simulink model "SecRwRtStLtwdRtwdTrgtPosSelc"  (R2018b)
settings: Solver=FixedStepDiscrete  StartTime=0.0  StopTime=10.0  FixedStep=0.01  RelTol=1e-3
undefined symbols (not defined in the file or in its folder): KeSMSw6sAcsEntrySecRwRtStLtwdRtwdPos_Val, KeSMSw6sAcsEntrySecRwRtStLtwdRtwdPosMax_Val, KeSMSw6sAcsEntrySecRwRtStLtwdRtwdPosMin_Val, KeSMSw6sAcsExtSecRwRtStLtwdRtwdPos_Val, KeSMSw6sAcsExtSecRwRtStLtwdRtwdPosMax_Val, KeSMSw6sAcsExtSecRwRtStLtwdRtwdPosMin_Val, KeSMSw6sFamilyMdSecRwRtStLtwdRtwdPos_Val, KeSMSw6sFamilyMdSecRwRtStLtwdRtwdPosMax_Val, KeSMSw6sFamilyMdSecRwRtStLtwdRtwdPosMin_Val, KeSMSw6sFamilyRMdSecRwRtStLtwdRtwdPos_Val, KeSMSw6sFamilyRMdSecRwRtStLtwdRtwdPosMax_Val, KeSMSw6sFamilyRMdSecRwRtStLtwdRtwdPosMin_Val, KeSMSw6sIntimacyMdSecRwRtStLtwdRtwdPos_Val, KeSMSw6sIntimacyMdSecRwRtStLtwdRtwdPosMax_Val, KeSMSw6sIntimacyMdSecRwRtStLtwdRtwdPosMin_Val, KeSMSw6sIntimacyRMdSecRwRtStLtwdRtwdPos_Val, KeSMSw6sIntimacyRMdSecRwRtStLtwdRtwdPosMax_Val, KeSMSw6sIntimacyRMdSecRwRtStLtwdRtwdPosMin_Val, KeSMSw6sVIPSecRwRtStLtwdRtwdPos_Val, KeSMSw6sVIPSecRwRtStLtwdRtwdPosMax_Val, KeSMSw6sVIPSecRwRtStLtwdRtwdPosMin_Val, KeSMSwAcsEntrySecRwRtStLtwdRtwdPos_Val, KeSMSwAcsEntrySecRwRtStLtwdRtwdPosMax_Val, KeSMSwAcsEntrySecRwRtStLtwdRtwdPosMin_Val, KeSMSwAcsExtSecRwRtStLtwdRtwdPos_Val, KeSMSwAcsExtSecRwRtStLtwdRtwdPosMax_Val, KeSMSwAcsExtSecRwRtStLtwdRtwdPosMin_Val, KeSMSwFamilyMdSecRwRtStLtwdRtwdPos_Val, KeSMSwFamilyMdSecRwRtStLtwdRtwdPosMax_Val, KeSMSwFamilyMdSecRwRtStLtwdRtwdPosMin_Val, KeSMSwFamilyRMdSecRwRtStLtwdRtwdPos_Val, KeSMSwFamilyRMdSecRwRtStLtwdRtwdPosMax_Val, KeSMSwFamilyRMdSecRwRtStLtwdRtwdPosMin_Val, KeSMSwIntimacyMdSecRwRtStLtwdRtwdPos_Val, KeSMSwIntimacyMdSecRwRtStLtwdRtwdPosMax_Val, KeSMSwIntimacyMdSecRwRtStLtwdRtwdPosMin_Val, KeSMSwIntimacyRMdSecRwRtStLtwdRtwdPos_Val, KeSMSwIntimacyRMdSecRwRtStLtwdRtwdPosMax_Val, KeSMSwIntimacyRMdSecRwRtStLtwdRtwdPosMin_Val, KeSMSwVIPSecRwRtStLtwdRtwdPos_Val, KeSMSwVIPSecRwRtStLtwdRtwdPosMax_Val, KeSMSwVIPSecRwRtStLtwdRtwdPosMin_Val
libraries: TrgtPosSelcLib x8
settings Model: Creator=sn2xws  LastModifiedBy=sn2xws
settings DataIOCC: SaveFormat=StructureWithTime
settings OptimizationCC: DefaultParameterBehavior=Inlined  EnhancedBackFolding=on  PassReuseOutputArgsAs=Individual arguments  ZeroExternalMemoryAtStartup=off  ZeroInternalMemoryAtStartup=off  OptimizeBlockOrder=speed  DifferentSizesBufferReuse=on  OptimizationCustomize=off
settings DebuggingCC: ParameterTunabilityLossMsg=error
settings ModelReferenceCC: ModelReferenceNumInstancesAllowed=Single
settings SFSimCC: MATLABDynamicMemAlloc=off
settings RTWCC: SystemTargetFile=autosar.tlc  GenCodeOnly=on  TemplateMakefile=ert_default_tmf  Description=AUTOSAR  GenerateReport=on  IncludeHyperlinkInReport=on  LaunchReport=on  GenerateTraceInfo=on  GenerateTraceReport=on  GenerateTraceReportSl=on  GenerateTraceReportSf=on  GenerateTraceReportEml=on
settings CodeAppCC: ForceParamTrailComments=on  IgnoreCustomStorageClasses=off  OperatorAnnotations=on  SimulinkDataObjDesc=on  SFDataObjDesc=on  InsertBlockDesc=on
settings STFCustomTargetCC: TargetLangStandard=C99 (ISO)  MultiwordLength=256  ParMdlRefBuildCompliant=on  CompOptLevelCompliant=on  IncludeMdlTerminateFcn=off  CombineOutputUpdateFcns=on  SuppressErrorStatus=on  ERTCustomFileBanners=on  SupportNonFinite=off  SupportComplex=off  SupportContinuousTime=off  SupportNonInlinedSFcns=off  RemoveResetFunc=on  MATLABClassNameForMDSCustomization=Simulink.SoftwareTarget.ERTCustomization  AutosarCompliant=on  UseToolchainInfoCompliant=on  LookupTableObjectStructAxisOrder=2,1,3,4,...  LUTObjectStructOrderEvenSpacing=Size,Table,Breakpoints  SystemTargetFile=autosar.tlc
settings ERTTargetCC: TargetLangStandard=C99 (ISO)  ConcurrentExecutionCompliant=off  IncludeMdlTerminateFcn=off  SuppressErrorStatus=on  SupportNonFinite=off  SupportComplex=off  ModelStepFunctionPrototypeControlCompliant=off  CPPClassGenCompliant=off  AutosarCompliant=on  LookupTableObjectStructAxisOrder=2,1,3,4,...  LUTObjectStructOrderEvenSpacing=Size,Table,Breakpoints  InlinedParameterPlacement=NonHierarchical  ERTCustomFileTemplate=example_file_process.tlc  ERTFilePackagingFormat=Compact

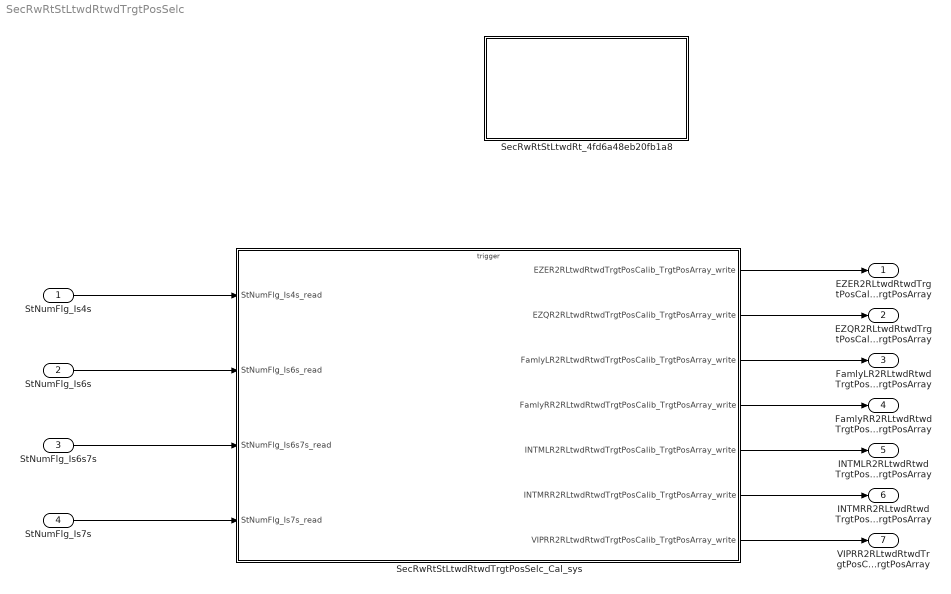
== system SecRwRtStLtwdRtwdTrgtPosSelc ==
  StNumFlg_Is4s : Inport  OutDataTypeStr=boolean  PortDimensions=1
  StNumFlg_Is6s : Inport  Port=2  OutDataTypeStr=boolean  PortDimensions=1
  StNumFlg_Is6s7s : Inport  Port=3  OutDataTypeStr=boolean  PortDimensions=1
  StNumFlg_Is7s : Inport  Port=4  OutDataTypeStr=boolean  PortDimensions=1
  SecRwRtStLtwdRt_4fd6a48eb20fb1a8 : Subsystem
  SecRwRtStLtwdRtwdTrgtPosSelc_Cal_sys : Subsystem
  EZER2RLtwdRtwdTrgtPosCalib_TrgtPosArray : Outport  Description=|  OutDataTypeStr=uint16  PortDimensions=3
      | 0:Pos
      | 1:Max
      | 2:Min
  EZQR2RLtwdRtwdTrgtPosCalib_TrgtPosArray : Outport  Description=|  Port=2  OutDataTypeStr=uint16  PortDimensions=3
      | 0:Pos
      | 1:Max
      | 2:Min
  FamlyLR2RLtwdRtwdTrgtPosCalib_TrgtPosArray : Outport  Description=|  Port=3  OutDataTypeStr=uint16  PortDimensions=3
      | 0:Pos
      | 1:Max
      | 2:Min
  FamlyRR2RLtwdRtwdTrgtPosCalib_TrgtPosArray : Outport  Description=|  Port=4  OutDataTypeStr=uint16  PortDimensions=3
      | 0:Pos
      | 1:Max
      | 2:Min
  INTMLR2RLtwdRtwdTrgtPosCalib_TrgtPosArray : Outport  Description=|  Port=5  OutDataTypeStr=uint16  PortDimensions=3
      | 0:Pos
      | 1:Max
      | 2:Min
  INTMRR2RLtwdRtwdTrgtPosCalib_TrgtPosArray : Outport  Description=|  Port=6  OutDataTypeStr=uint16  PortDimensions=3
      | 0:Pos
      | 1:Max
      | 2:Min
  VIPRR2RLtwdRtwdTrgtPosCalib_TrgtPosArray : Outport  Description=|  Port=7  OutDataTypeStr=uint16  PortDimensions=3
      | 0:Pos
      | 1:Max
      | 2:Min
  wires:
  StNumFlg_Is4s/1 -> SecRwRtStLtwdRtwdTrgtPosSelc_Cal_sys/1(StNumFlg_Is4s_read)
  StNumFlg_Is6s/1 -> SecRwRtStLtwdRtwdTrgtPosSelc_Cal_sys/2(StNumFlg_Is6s_read)
  StNumFlg_Is6s7s/1 -> SecRwRtStLtwdRtwdTrgtPosSelc_Cal_sys/3(StNumFlg_Is6s7s_read)
  StNumFlg_Is7s/1 -> SecRwRtStLtwdRtwdTrgtPosSelc_Cal_sys/4(StNumFlg_Is7s_read)
  SecRwRtStLtwdRtwdTrgtPosSelc_Cal_sys/1(EZER2RLtwdRtwdTrgtPosCalib_TrgtPosArray_write) -> EZER2RLtwdRtwdTrgtPosCalib_TrgtPosArray/1
  SecRwRtStLtwdRtwdTrgtPosSelc_Cal_sys/2(EZQR2RLtwdRtwdTrgtPosCalib_TrgtPosArray_write) -> EZQR2RLtwdRtwdTrgtPosCalib_TrgtPosArray/1
  SecRwRtStLtwdRtwdTrgtPosSelc_Cal_sys/3(FamlyLR2RLtwdRtwdTrgtPosCalib_TrgtPosArray_write) -> FamlyLR2RLtwdRtwdTrgtPosCalib_TrgtPosArray/1
  SecRwRtStLtwdRtwdTrgtPosSelc_Cal_sys/4(FamlyRR2RLtwdRtwdTrgtPosCalib_TrgtPosArray_write) -> FamlyRR2RLtwdRtwdTrgtPosCalib_TrgtPosArray/1
  SecRwRtStLtwdRtwdTrgtPosSelc_Cal_sys/5(INTMLR2RLtwdRtwdTrgtPosCalib_TrgtPosArray_write) -> INTMLR2RLtwdRtwdTrgtPosCalib_TrgtPosArray/1
  SecRwRtStLtwdRtwdTrgtPosSelc_Cal_sys/6(INTMRR2RLtwdRtwdTrgtPosCalib_TrgtPosArray_write) -> INTMRR2RLtwdRtwdTrgtPosCalib_TrgtPosArray/1
  SecRwRtStLtwdRtwdTrgtPosSelc_Cal_sys/7(VIPRR2RLtwdRtwdTrgtPosCalib_TrgtPosArray_write) -> VIPRR2RLtwdRtwdTrgtPosCalib_TrgtPosArray/1

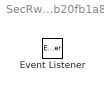
== system SecRwRtStLtwdRtwdTrgtPosSelc/SecRwRtStLtwdRt_4fd6a48eb20fb1a8 ==
  Event Listener : EventListener  EventName=reset

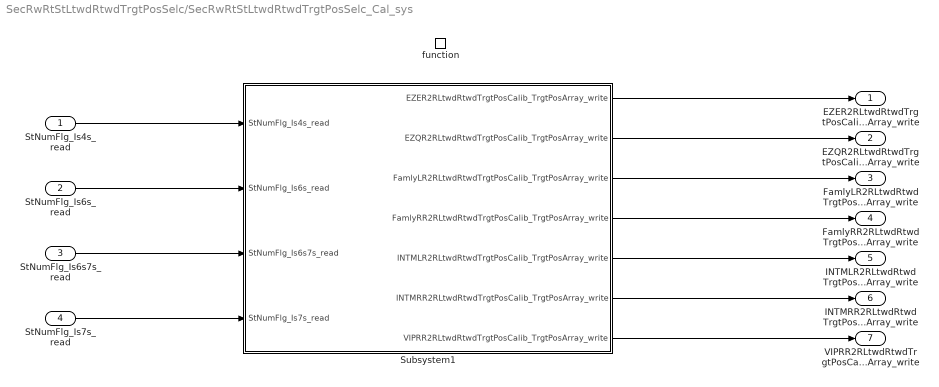
== system SecRwRtStLtwdRtwdTrgtPosSelc/SecRwRtStLtwdRtwdTrgtPosSelc_Cal_sys ==
  StNumFlg_Is4s_read : Inport
  StNumFlg_Is6s_read : Inport  Port=2
  StNumFlg_Is6s7s_read : Inport  Port=3
  StNumFlg_Is7s_read : Inport  Port=4
  function : TriggerPort  TriggerType=function-call  IsSimulinkFunction=on  FunctionName=SecRwRtStLtwdRtwdTrgtPosSelc_Cal  VariantControl=(inherit)
  Subsystem1 : Subsystem
  EZER2RLtwdRtwdTrgtPosCalib_TrgtPosArray_write : Outport
      settings: EnsureOutportIsVirtual=on
  EZQR2RLtwdRtwdTrgtPosCalib_TrgtPosArray_write : Outport  Port=2
      settings: EnsureOutportIsVirtual=on
  FamlyLR2RLtwdRtwdTrgtPosCalib_TrgtPosArray_write : Outport  Port=3
      settings: EnsureOutportIsVirtual=on
  FamlyRR2RLtwdRtwdTrgtPosCalib_TrgtPosArray_write : Outport  Port=4
      settings: EnsureOutportIsVirtual=on
  INTMLR2RLtwdRtwdTrgtPosCalib_TrgtPosArray_write : Outport  Port=5
      settings: EnsureOutportIsVirtual=on
  INTMRR2RLtwdRtwdTrgtPosCalib_TrgtPosArray_write : Outport  Port=6
      settings: EnsureOutportIsVirtual=on
  VIPRR2RLtwdRtwdTrgtPosCalib_TrgtPosArray_write : Outport  Port=7
      settings: EnsureOutportIsVirtual=on
  wires:
  Subsystem1/1(EZER2RLtwdRtwdTrgtPosCalib_TrgtPosArray_write) -> EZER2RLtwdRtwdTrgtPosCalib_TrgtPosArray_write/1
  Subsystem1/2(EZQR2RLtwdRtwdTrgtPosCalib_TrgtPosArray_write) -> EZQR2RLtwdRtwdTrgtPosCalib_TrgtPosArray_write/1
  Subsystem1/3(FamlyLR2RLtwdRtwdTrgtPosCalib_TrgtPosArray_write) -> FamlyLR2RLtwdRtwdTrgtPosCalib_TrgtPosArray_write/1
  Subsystem1/4(FamlyRR2RLtwdRtwdTrgtPosCalib_TrgtPosArray_write) -> FamlyRR2RLtwdRtwdTrgtPosCalib_TrgtPosArray_write/1
  Subsystem1/5(INTMLR2RLtwdRtwdTrgtPosCalib_TrgtPosArray_write) -> INTMLR2RLtwdRtwdTrgtPosCalib_TrgtPosArray_write/1
  Subsystem1/6(INTMRR2RLtwdRtwdTrgtPosCalib_TrgtPosArray_write) -> INTMRR2RLtwdRtwdTrgtPosCalib_TrgtPosArray_write/1
  Subsystem1/7(VIPRR2RLtwdRtwdTrgtPosCalib_TrgtPosArray_write) -> VIPRR2RLtwdRtwdTrgtPosCalib_TrgtPosArray_write/1
  StNumFlg_Is4s_read/1 -> Subsystem1/1(StNumFlg_Is4s_read)
  StNumFlg_Is6s_read/1 -> Subsystem1/2(StNumFlg_Is6s_read)
  StNumFlg_Is6s7s_read/1 -> Subsystem1/3(StNumFlg_Is6s7s_read)
  StNumFlg_Is7s_read/1 -> Subsystem1/4(StNumFlg_Is7s_read)

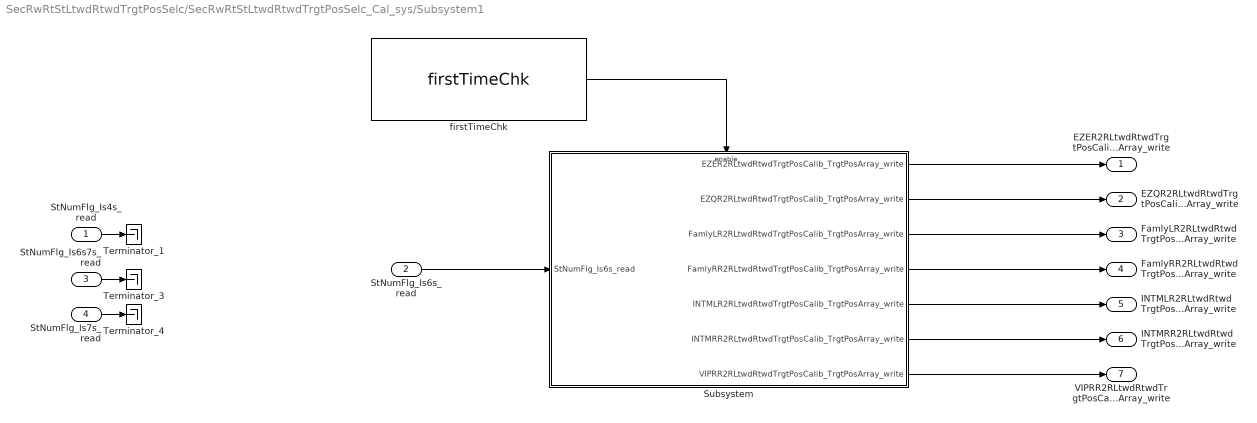
== system SecRwRtStLtwdRtwdTrgtPosSelc/SecRwRtStLtwdRtwdTrgtPosSelc_Cal_sys/Subsystem1 ==
  StNumFlg_Is4s_read : Inport
  StNumFlg_Is6s_read : Inport  Port=2
  StNumFlg_Is6s7s_read : Inport  Port=3
  StNumFlg_Is7s_read : Inport  Port=4
  Subsystem : Subsystem
  Terminator_1 : Terminator
  Terminator_3 : Terminator
  Terminator_4 : Terminator
  firstTimeChk : TrgtPosSelcLib/firstTimeChk  SystemSampleTime=-1
  EZER2RLtwdRtwdTrgtPosCalib_TrgtPosArray_write : Outport
      settings: EnsureOutportIsVirtual=on
  EZQR2RLtwdRtwdTrgtPosCalib_TrgtPosArray_write : Outport  Port=2
      settings: EnsureOutportIsVirtual=on
  FamlyLR2RLtwdRtwdTrgtPosCalib_TrgtPosArray_write : Outport  Port=3
      settings: EnsureOutportIsVirtual=on
  FamlyRR2RLtwdRtwdTrgtPosCalib_TrgtPosArray_write : Outport  Port=4
      settings: EnsureOutportIsVirtual=on
  INTMLR2RLtwdRtwdTrgtPosCalib_TrgtPosArray_write : Outport  Port=5
      settings: EnsureOutportIsVirtual=on
  INTMRR2RLtwdRtwdTrgtPosCalib_TrgtPosArray_write : Outport  Port=6
      settings: EnsureOutportIsVirtual=on
  VIPRR2RLtwdRtwdTrgtPosCalib_TrgtPosArray_write : Outport  Port=7
      settings: EnsureOutportIsVirtual=on
  wires:
  Subsystem/2(EZQR2RLtwdRtwdTrgtPosCalib_TrgtPosArray_write) -> EZQR2RLtwdRtwdTrgtPosCalib_TrgtPosArray_write/1
  StNumFlg_Is6s_read/1 -> Subsystem/1(StNumFlg_Is6s_read)
  StNumFlg_Is6s7s_read/1 -> Terminator_3/1
  firstTimeChk/1 -> Subsystem/Enable
  Subsystem/1(EZER2RLtwdRtwdTrgtPosCalib_TrgtPosArray_write) -> EZER2RLtwdRtwdTrgtPosCalib_TrgtPosArray_write/1
  StNumFlg_Is7s_read/1 -> Terminator_4/1
  Subsystem/3(FamlyLR2RLtwdRtwdTrgtPosCalib_TrgtPosArray_write) -> FamlyLR2RLtwdRtwdTrgtPosCalib_TrgtPosArray_write/1
  Subsystem/4(FamlyRR2RLtwdRtwdTrgtPosCalib_TrgtPosArray_write) -> FamlyRR2RLtwdRtwdTrgtPosCalib_TrgtPosArray_write/1
  Subsystem/5(INTMLR2RLtwdRtwdTrgtPosCalib_TrgtPosArray_write) -> INTMLR2RLtwdRtwdTrgtPosCalib_TrgtPosArray_write/1
  Subsystem/7(VIPRR2RLtwdRtwdTrgtPosCalib_TrgtPosArray_write) -> VIPRR2RLtwdRtwdTrgtPosCalib_TrgtPosArray_write/1
  StNumFlg_Is4s_read/1 -> Terminator_1/1
  Subsystem/6(INTMRR2RLtwdRtwdTrgtPosCalib_TrgtPosArray_write) -> INTMRR2RLtwdRtwdTrgtPosCalib_TrgtPosArray_write/1

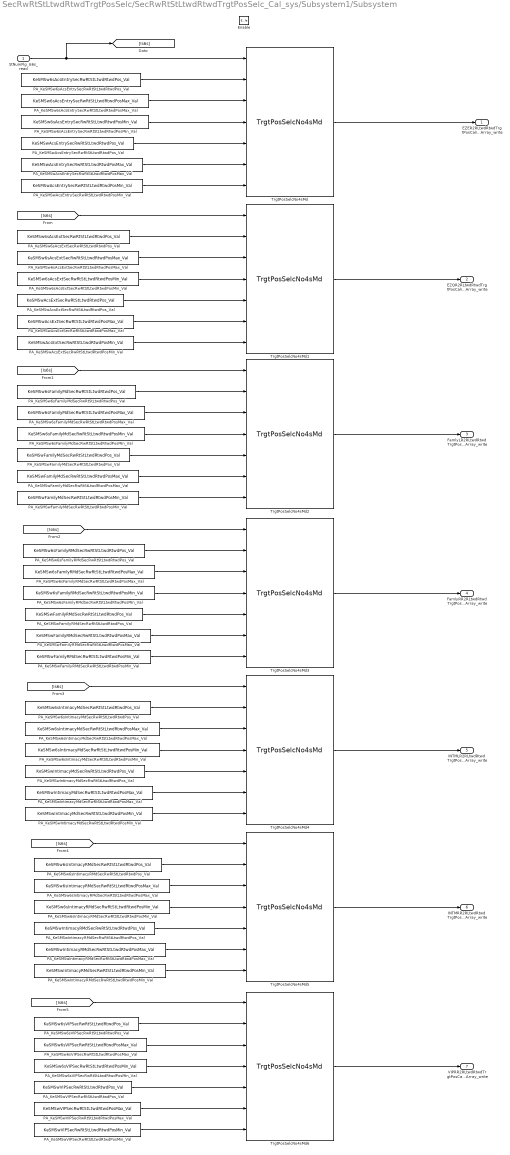
== system SecRwRtStLtwdRtwdTrgtPosSelc/SecRwRtStLtwdRtwdTrgtPosSelc_Cal_sys/Subsystem1/Subsystem ==
  StNumFlg_Is6s_read : Inport
  Enable : EnablePort
  PA_KeSMSw6sAcsEntrySecRwRtStLtwdRtwdPosMax_Val : Constant  Value=KeSMSw6sAcsEntrySecRwRtStLtwdRtwdPosMax_Val
  PA_KeSMSw6sAcsEntrySecRwRtStLtwdRtwdPosMin_Val : Constant  Value=KeSMSw6sAcsEntrySecRwRtStLtwdRtwdPosMin_Val
  PA_KeSMSw6sAcsEntrySecRwRtStLtwdRtwdPos_Val : Constant  Value=KeSMSw6sAcsEntrySecRwRtStLtwdRtwdPos_Val
  PA_KeSMSw6sAcsExtSecRwRtStLtwdRtwdPosMax_Val : Constant  Value=KeSMSw6sAcsExtSecRwRtStLtwdRtwdPosMax_Val
  PA_KeSMSw6sAcsExtSecRwRtStLtwdRtwdPosMin_Val : Constant  Value=KeSMSw6sAcsExtSecRwRtStLtwdRtwdPosMin_Val
  PA_KeSMSw6sAcsExtSecRwRtStLtwdRtwdPos_Val : Constant  Value=KeSMSw6sAcsExtSecRwRtStLtwdRtwdPos_Val
  PA_KeSMSw6sFamilyMdSecRwRtStLtwdRtwdPosMax_Val : Constant  Value=KeSMSw6sFamilyMdSecRwRtStLtwdRtwdPosMax_Val
  PA_KeSMSw6sFamilyMdSecRwRtStLtwdRtwdPosMin_Val : Constant  Value=KeSMSw6sFamilyMdSecRwRtStLtwdRtwdPosMin_Val
  PA_KeSMSw6sFamilyMdSecRwRtStLtwdRtwdPos_Val : Constant  Value=KeSMSw6sFamilyMdSecRwRtStLtwdRtwdPos_Val
  PA_KeSMSw6sFamilyRMdSecRwRtStLtwdRtwdPosMax_Val : Constant  Value=KeSMSw6sFamilyRMdSecRwRtStLtwdRtwdPosMax_Val
  PA_KeSMSw6sFamilyRMdSecRwRtStLtwdRtwdPosMin_Val : Constant  Value=KeSMSw6sFamilyRMdSecRwRtStLtwdRtwdPosMin_Val
  PA_KeSMSw6sFamilyRMdSecRwRtStLtwdRtwdPos_Val : Constant  Value=KeSMSw6sFamilyRMdSecRwRtStLtwdRtwdPos_Val
  PA_KeSMSw6sIntimacyMdSecRwRtStLtwdRtwdPosMax_Val : Constant  Value=KeSMSw6sIntimacyMdSecRwRtStLtwdRtwdPosMax_Val
  PA_KeSMSw6sIntimacyMdSecRwRtStLtwdRtwdPosMin_Val : Constant  Value=KeSMSw6sIntimacyMdSecRwRtStLtwdRtwdPosMin_Val
  PA_KeSMSw6sIntimacyMdSecRwRtStLtwdRtwdPos_Val : Constant  Value=KeSMSw6sIntimacyMdSecRwRtStLtwdRtwdPos_Val
  PA_KeSMSw6sIntimacyRMdSecRwRtStLtwdRtwdPosMax_Val : Constant  Value=KeSMSw6sIntimacyRMdSecRwRtStLtwdRtwdPosMax_Val
  PA_KeSMSw6sIntimacyRMdSecRwRtStLtwdRtwdPosMin_Val : Constant  Value=KeSMSw6sIntimacyRMdSecRwRtStLtwdRtwdPosMin_Val
  PA_KeSMSw6sIntimacyRMdSecRwRtStLtwdRtwdPos_Val : Constant  Value=KeSMSw6sIntimacyRMdSecRwRtStLtwdRtwdPos_Val
  PA_KeSMSw6sVIPSecRwRtStLtwdRtwdPosMax_Val : Constant  Value=KeSMSw6sVIPSecRwRtStLtwdRtwdPosMax_Val
  PA_KeSMSw6sVIPSecRwRtStLtwdRtwdPosMin_Val : Constant  Value=KeSMSw6sVIPSecRwRtStLtwdRtwdPosMin_Val
  PA_KeSMSw6sVIPSecRwRtStLtwdRtwdPos_Val : Constant  Value=KeSMSw6sVIPSecRwRtStLtwdRtwdPos_Val
  PA_KeSMSwAcsEntrySecRwRtStLtwdRtwdPosMax_Val : Constant  Value=KeSMSwAcsEntrySecRwRtStLtwdRtwdPosMax_Val
  PA_KeSMSwAcsEntrySecRwRtStLtwdRtwdPosMin_Val : Constant  Value=KeSMSwAcsEntrySecRwRtStLtwdRtwdPosMin_Val
  PA_KeSMSwAcsEntrySecRwRtStLtwdRtwdPos_Val : Constant  Value=KeSMSwAcsEntrySecRwRtStLtwdRtwdPos_Val
  PA_KeSMSwAcsExtSecRwRtStLtwdRtwdPosMax_Val : Constant  Value=KeSMSwAcsExtSecRwRtStLtwdRtwdPosMax_Val
  PA_KeSMSwAcsExtSecRwRtStLtwdRtwdPosMin_Val : Constant  Value=KeSMSwAcsExtSecRwRtStLtwdRtwdPosMin_Val
  PA_KeSMSwAcsExtSecRwRtStLtwdRtwdPos_Val : Constant  Value=KeSMSwAcsExtSecRwRtStLtwdRtwdPos_Val
  PA_KeSMSwFamilyMdSecRwRtStLtwdRtwdPosMax_Val : Constant  Value=KeSMSwFamilyMdSecRwRtStLtwdRtwdPosMax_Val
  PA_KeSMSwFamilyMdSecRwRtStLtwdRtwdPosMin_Val : Constant  Value=KeSMSwFamilyMdSecRwRtStLtwdRtwdPosMin_Val
  PA_KeSMSwFamilyMdSecRwRtStLtwdRtwdPos_Val : Constant  Value=KeSMSwFamilyMdSecRwRtStLtwdRtwdPos_Val
  PA_KeSMSwFamilyRMdSecRwRtStLtwdRtwdPosMax_Val : Constant  Value=KeSMSwFamilyRMdSecRwRtStLtwdRtwdPosMax_Val
  PA_KeSMSwFamilyRMdSecRwRtStLtwdRtwdPosMin_Val : Constant  Value=KeSMSwFamilyRMdSecRwRtStLtwdRtwdPosMin_Val
  PA_KeSMSwFamilyRMdSecRwRtStLtwdRtwdPos_Val : Constant  Value=KeSMSwFamilyRMdSecRwRtStLtwdRtwdPos_Val
  PA_KeSMSwIntimacyMdSecRwRtStLtwdRtwdPosMax_Val : Constant  Value=KeSMSwIntimacyMdSecRwRtStLtwdRtwdPosMax_Val
  PA_KeSMSwIntimacyMdSecRwRtStLtwdRtwdPosMin_Val : Constant  Value=KeSMSwIntimacyMdSecRwRtStLtwdRtwdPosMin_Val
  PA_KeSMSwIntimacyMdSecRwRtStLtwdRtwdPos_Val : Constant  Value=KeSMSwIntimacyMdSecRwRtStLtwdRtwdPos_Val
  PA_KeSMSwIntimacyRMdSecRwRtStLtwdRtwdPosMax_Val : Constant  Value=KeSMSwIntimacyRMdSecRwRtStLtwdRtwdPosMax_Val
  PA_KeSMSwIntimacyRMdSecRwRtStLtwdRtwdPosMin_Val : Constant  Value=KeSMSwIntimacyRMdSecRwRtStLtwdRtwdPosMin_Val
  PA_KeSMSwIntimacyRMdSecRwRtStLtwdRtwdPos_Val : Constant  Value=KeSMSwIntimacyRMdSecRwRtStLtwdRtwdPos_Val
  PA_KeSMSwVIPSecRwRtStLtwdRtwdPosMax_Val : Constant  Value=KeSMSwVIPSecRwRtStLtwdRtwdPosMax_Val
  PA_KeSMSwVIPSecRwRtStLtwdRtwdPosMin_Val : Constant  Value=KeSMSwVIPSecRwRtStLtwdRtwdPosMin_Val
  PA_KeSMSwVIPSecRwRtStLtwdRtwdPos_Val : Constant  Value=KeSMSwVIPSecRwRtStLtwdRtwdPos_Val
  TrgtPosSelcNo4sMd{,1..6} (7 alike) : TrgtPosSelcLib/TrgtPosSelcNo4sMd  SystemSampleTime=-1
  EZER2RLtwdRtwdTrgtPosCalib_TrgtPosArray_write : Outport
      settings: EnsureOutportIsVirtual=on
  EZQR2RLtwdRtwdTrgtPosCalib_TrgtPosArray_write : Outport  Port=2
      settings: EnsureOutportIsVirtual=on
  FamlyLR2RLtwdRtwdTrgtPosCalib_TrgtPosArray_write : Outport  Port=3
      settings: EnsureOutportIsVirtual=on
  FamlyRR2RLtwdRtwdTrgtPosCalib_TrgtPosArray_write : Outport  Port=4
      settings: EnsureOutportIsVirtual=on
  INTMLR2RLtwdRtwdTrgtPosCalib_TrgtPosArray_write : Outport  Port=5
      settings: EnsureOutportIsVirtual=on
  INTMRR2RLtwdRtwdTrgtPosCalib_TrgtPosArray_write : Outport  Port=6
      settings: EnsureOutportIsVirtual=on
  VIPRR2RLtwdRtwdTrgtPosCalib_TrgtPosArray_write : Outport  Port=7
      settings: EnsureOutportIsVirtual=on
  wires:
  TrgtPosSelcNo4sMd/1 -> EZER2RLtwdRtwdTrgtPosCalib_TrgtPosArray_write/1
  TrgtPosSelcNo4sMd1/1 -> EZQR2RLtwdRtwdTrgtPosCalib_TrgtPosArray_write/1
  StNumFlg_Is6s_read/1 -> [Is6s], TrgtPosSelcNo4sMd/1
  [Is6s] -> TrgtPosSelcNo4sMd1/1
  [Is6s] -> TrgtPosSelcNo4sMd2/1
  [Is6s] -> TrgtPosSelcNo4sMd3/1
  [Is6s] -> TrgtPosSelcNo4sMd4/1
  [Is6s] -> TrgtPosSelcNo4sMd5/1
  [Is6s] -> TrgtPosSelcNo4sMd6/1
  TrgtPosSelcNo4sMd2/1 -> FamlyLR2RLtwdRtwdTrgtPosCalib_TrgtPosArray_write/1
  TrgtPosSelcNo4sMd3/1 -> FamlyRR2RLtwdRtwdTrgtPosCalib_TrgtPosArray_write/1
  TrgtPosSelcNo4sMd4/1 -> INTMLR2RLtwdRtwdTrgtPosCalib_TrgtPosArray_write/1
  TrgtPosSelcNo4sMd5/1 -> INTMRR2RLtwdRtwdTrgtPosCalib_TrgtPosArray_write/1
  TrgtPosSelcNo4sMd6/1 -> VIPRR2RLtwdRtwdTrgtPosCalib_TrgtPosArray_write/1
  PA_KeSMSw6sAcsEntrySecRwRtStLtwdRtwdPosMax_Val/1 -> TrgtPosSelcNo4sMd/3
  PA_KeSMSw6sAcsEntrySecRwRtStLtwdRtwdPos_Val/1 -> TrgtPosSelcNo4sMd/2
  PA_KeSMSw6sAcsEntrySecRwRtStLtwdRtwdPosMin_Val/1 -> TrgtPosSelcNo4sMd/4
  PA_KeSMSw6sAcsExtSecRwRtStLtwdRtwdPosMax_Val/1 -> TrgtPosSelcNo4sMd1/3
  PA_KeSMSw6sAcsExtSecRwRtStLtwdRtwdPos_Val/1 -> TrgtPosSelcNo4sMd1/2
  PA_KeSMSw6sAcsExtSecRwRtStLtwdRtwdPosMin_Val/1 -> TrgtPosSelcNo4sMd1/4
  PA_KeSMSw6sFamilyMdSecRwRtStLtwdRtwdPosMax_Val/1 -> TrgtPosSelcNo4sMd2/3
  PA_KeSMSw6sFamilyMdSecRwRtStLtwdRtwdPos_Val/1 -> TrgtPosSelcNo4sMd2/2
  PA_KeSMSw6sFamilyMdSecRwRtStLtwdRtwdPosMin_Val/1 -> TrgtPosSelcNo4sMd2/4
  PA_KeSMSw6sFamilyRMdSecRwRtStLtwdRtwdPosMax_Val/1 -> TrgtPosSelcNo4sMd3/3
  PA_KeSMSw6sFamilyRMdSecRwRtStLtwdRtwdPos_Val/1 -> TrgtPosSelcNo4sMd3/2
  PA_KeSMSw6sFamilyRMdSecRwRtStLtwdRtwdPosMin_Val/1 -> TrgtPosSelcNo4sMd3/4
  PA_KeSMSw6sIntimacyMdSecRwRtStLtwdRtwdPosMax_Val/1 -> TrgtPosSelcNo4sMd4/3
  PA_KeSMSw6sIntimacyMdSecRwRtStLtwdRtwdPosMin_Val/1 -> TrgtPosSelcNo4sMd4/4
  PA_KeSMSw6sIntimacyMdSecRwRtStLtwdRtwdPos_Val/1 -> TrgtPosSelcNo4sMd4/2
  PA_KeSMSw6sIntimacyRMdSecRwRtStLtwdRtwdPosMin_Val/1 -> TrgtPosSelcNo4sMd5/4
  PA_KeSMSw6sIntimacyRMdSecRwRtStLtwdRtwdPosMax_Val/1 -> TrgtPosSelcNo4sMd5/3
  PA_KeSMSw6sIntimacyRMdSecRwRtStLtwdRtwdPos_Val/1 -> TrgtPosSelcNo4sMd5/2
  PA_KeSMSw6sVIPSecRwRtStLtwdRtwdPosMax_Val/1 -> TrgtPosSelcNo4sMd6/3
  PA_KeSMSw6sVIPSecRwRtStLtwdRtwdPos_Val/1 -> TrgtPosSelcNo4sMd6/2
  PA_KeSMSw6sVIPSecRwRtStLtwdRtwdPosMin_Val/1 -> TrgtPosSelcNo4sMd6/4
  PA_KeSMSwAcsEntrySecRwRtStLtwdRtwdPosMax_Val/1 -> TrgtPosSelcNo4sMd/6
  PA_KeSMSwAcsEntrySecRwRtStLtwdRtwdPos_Val/1 -> TrgtPosSelcNo4sMd/5
  PA_KeSMSwAcsEntrySecRwRtStLtwdRtwdPosMin_Val/1 -> TrgtPosSelcNo4sMd/7
  PA_KeSMSwAcsExtSecRwRtStLtwdRtwdPosMax_Val/1 -> TrgtPosSelcNo4sMd1/6
  PA_KeSMSwAcsExtSecRwRtStLtwdRtwdPosMin_Val/1 -> TrgtPosSelcNo4sMd1/7
  PA_KeSMSwAcsExtSecRwRtStLtwdRtwdPos_Val/1 -> TrgtPosSelcNo4sMd1/5
  PA_KeSMSwFamilyMdSecRwRtStLtwdRtwdPosMax_Val/1 -> TrgtPosSelcNo4sMd2/6
  PA_KeSMSwFamilyMdSecRwRtStLtwdRtwdPosMin_Val/1 -> TrgtPosSelcNo4sMd2/7
  PA_KeSMSwFamilyMdSecRwRtStLtwdRtwdPos_Val/1 -> TrgtPosSelcNo4sMd2/5
  PA_KeSMSwFamilyRMdSecRwRtStLtwdRtwdPosMax_Val/1 -> TrgtPosSelcNo4sMd3/6
  PA_KeSMSwFamilyRMdSecRwRtStLtwdRtwdPos_Val/1 -> TrgtPosSelcNo4sMd3/5
  PA_KeSMSwFamilyRMdSecRwRtStLtwdRtwdPosMin_Val/1 -> TrgtPosSelcNo4sMd3/7
  PA_KeSMSwIntimacyMdSecRwRtStLtwdRtwdPosMax_Val/1 -> TrgtPosSelcNo4sMd4/6
  PA_KeSMSwIntimacyMdSecRwRtStLtwdRtwdPosMin_Val/1 -> TrgtPosSelcNo4sMd4/7
  PA_KeSMSwIntimacyMdSecRwRtStLtwdRtwdPos_Val/1 -> TrgtPosSelcNo4sMd4/5
  PA_KeSMSwIntimacyRMdSecRwRtStLtwdRtwdPosMax_Val/1 -> TrgtPosSelcNo4sMd5/6
  PA_KeSMSwIntimacyRMdSecRwRtStLtwdRtwdPosMin_Val/1 -> TrgtPosSelcNo4sMd5/7
  PA_KeSMSwIntimacyRMdSecRwRtStLtwdRtwdPos_Val/1 -> TrgtPosSelcNo4sMd5/5
  PA_KeSMSwVIPSecRwRtStLtwdRtwdPosMax_Val/1 -> TrgtPosSelcNo4sMd6/6
  PA_KeSMSwVIPSecRwRtStLtwdRtwdPos_Val/1 -> TrgtPosSelcNo4sMd6/5
  PA_KeSMSwVIPSecRwRtStLtwdRtwdPosMin_Val/1 -> TrgtPosSelcNo4sMd6/7
